simulink model "logisticregression"  (R2017a)
settings: Solver=FixedStepDiscrete  StartTime=0.0  StopTime=Inf  FixedStep=0.01  RelTol=1e-3  EnableMultiTasking=on
undefined symbols (not defined in the file or in its folder): DiscIntNeverNeededParam
libraries: autodiff x8
settings Model: Creator=eruffaldi  LastModifiedBy=eruffaldi
settings OptimizationCC: LifeSpan=inf
settings DebuggingCC: SFUnexpectedBacktrackingDiag=warning  SFNoUnconditionalDefaultTransitionDiag=warning  SFExecutionAtInitializationDiag=none
settings GRTTargetCC: TargetLangStandard=C89/C90 (ANSI)  GeneratePreprocessorConditionals=Disable all
settings ConfigComp: CovMetricSettings=dw  CovHtmlReporting=on  CovSaveCumulativeToWorkspaceVar=on  CovSaveSingleToWorkspaceVar=on  CovExternalEMLEnable=off

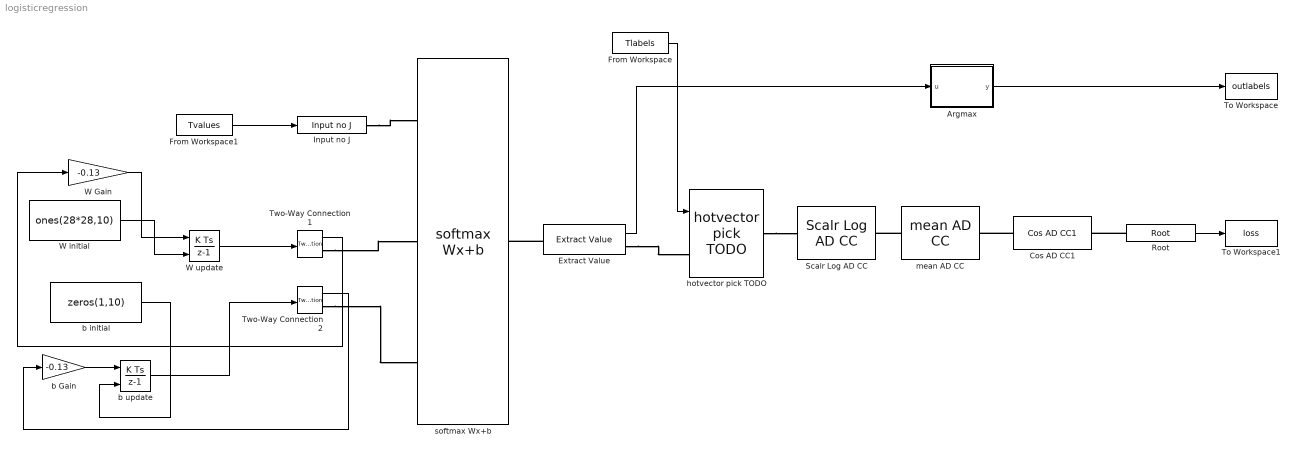
== system logisticregression ==
  Argmax : MATLAB Function  TreatAsAtomicUnit=on  mask{dim=1}
      mask prompts: dim "Dimension"
  Cos AD CC1 : autodiff/Cos AD CC1  gain=-1
      settings: SourceProductName=AutoDiff
  Extract Value : autodiff/Extract Value  SystemSampleTime=-1
      settings: SourceProductName=AutoDiff
  From Workspace : FromWorkspace  VariableName=Tlabels  SampleTime=0
  From Workspace1 : FromWorkspace  VariableName=Tvalues  SampleTime=0
  Input no J : autodiff/Input no J  SystemSampleTime=-1
      settings: SourceProductName=AutoDiff
  Root : autodiff/Root  SystemSampleTime=-1
      settings: SourceProductName=AutoDiff
  Scalr Log AD CC : autodiff/Scalr Log AD CC  SystemSampleTime=-1
      settings: SourceProductName=AutoDiff
  To Workspace : ToWorkspace  VariableName=outlabels  SaveFormat=Timeseries  SampleTime=-1
  To Workspace1 : ToWorkspace  VariableName=loss  SaveFormat=Timeseries  SampleTime=-1
  Two-Way Connection1 : TwoWayConnection
  Two-Way Connection2 : TwoWayConnection
  W Gain : Gain  Gain=-0.13
  W initial : Constant  Value=ones(28*28,10)
  W update : DiscreteIntegrator  InitialConditionSource=external  InitialConditionSetting=State (most efficient)  SampleTime=-1  ICPrevOutput=DiscIntNeverNeededParam  ICPrevScaledInput=DiscIntNeverNeededParam
  b Gain : Gain  Gain=-0.13
  b initial : Constant  Value=zeros(1,10)
  b update : DiscreteIntegrator  InitialConditionSource=external  InitialConditionSetting=State (most efficient)  SampleTime=-1  ICPrevOutput=DiscIntNeverNeededParam  ICPrevScaledInput=DiscIntNeverNeededParam
  hotvector pick TODO : autodiff/hotvector pick TODO
      settings: SourceProductName=AutoDiff
  mean AD CC : autodiff/mean AD CC
      settings: SourceProductName=AutoDiff
  softmax Wx+b : autodiff/softmax Wx+b
      settings: SourceProductName=AutoDiff
  wires:
  W initial/1 -> W update/2
  Two-Way Connection1/1 -> W Gain/1
  b initial/1 -> b update/2
  Two-Way Connection2/1 -> b Gain/1
  W Gain/1 -> W update/1
  b Gain/1 -> b update/1
  Argmax/1(y) -> To Workspace/1
  From Workspace1/1 -> Input no J/1
  W update/1 -> Two-Way Connection1/1
  b update/1 -> Two-Way Connection2/1
  Extract Value/1 -> Argmax/1(u)
  Root/1 -> To Workspace1/1
  From Workspace/1 -> hotvector pick TODO/1
  connections:
  mean AD CC/LConn1 -- Scalr Log AD CC/RConn1
  Two-Way Connection1/RConn1 -- softmax Wx+b/LConn2
  Two-Way Connection2/RConn1 -- softmax Wx+b/LConn3
  Input no J/RConn1 -- softmax Wx+b/LConn1
  Extract Value/LConn1 -- softmax Wx+b/RConn1
  Root/LConn1 -- Cos AD CC1/RConn1
  Cos AD CC1/LConn1 -- mean AD CC/RConn1
  hotvector pick TODO/RConn1 -- Scalr Log AD CC/LConn1
  Extract Value/RConn1 -- hotvector pick TODO/LConn1

== matlab function logisticregression/Argmax ==
  data: u input; y output
function y = fcn(u)

[~,y] = min(u,[],dim);
